simulink model "deney6"  (R2023b)
settings: Solver=VariableStepAuto  StartTime=0.0  StopTime=0.08  RelTol=1e-3
libraries: dspfdesign x1, commrandsrc3 x1, spsDiscreteVariableTimeDelayLib x1, commsink2 x1, commutil2 x1
settings Model: Creator=fatih  LastModifiedBy=fatih

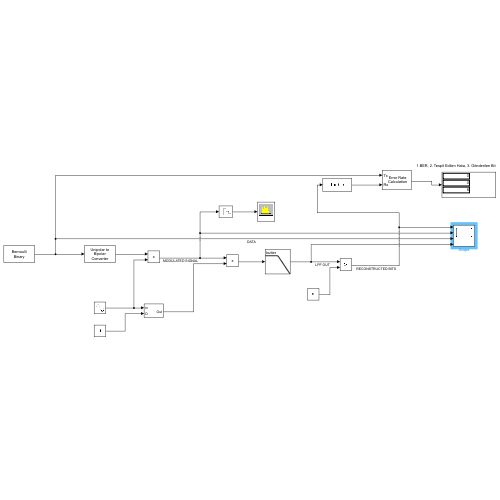
[thumbnail: Simulink's stored preview of the top-level diagram]
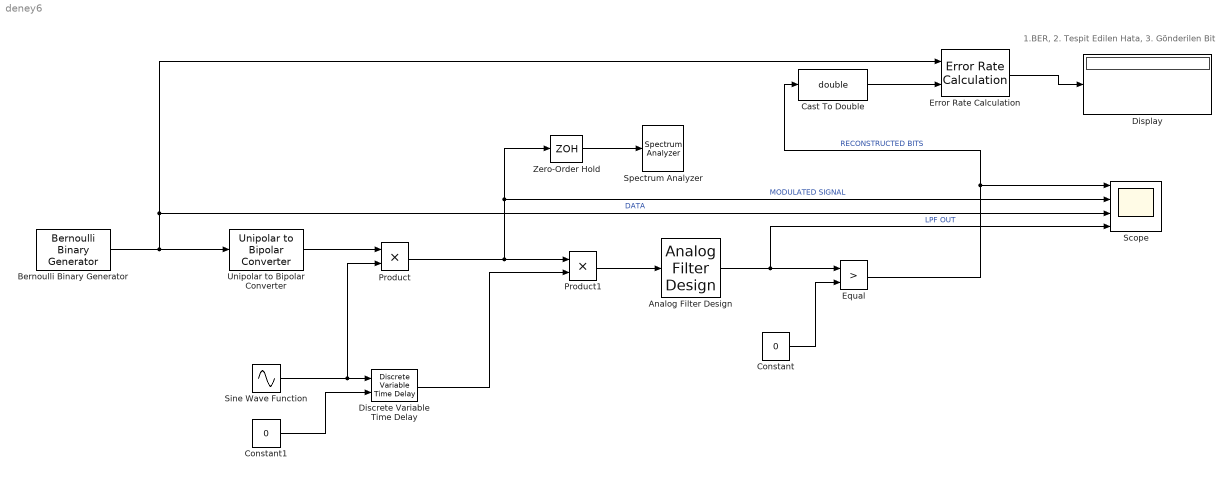
== system deney6 ==
  note: 1.BER, 2. Tespit Edilen Hata, 3. Gönderilen Bit
  Analog Filter Design : dspfdesign/Analog Filter Design  method=Butterworth  filttype=Lowpass  N=8  Wlo=2*pi*100  Whi=80  Rp=2  Rs=40
  Bernoulli Binary Generator : commrandsrc3/Bernoulli Binary Generator  ProbabilityOfZero=0.5  SeedSource=Auto  Seed=0  SampleTime=0.01  SamplesPerFrame=1  OutputDataType=double  SimulateUsing=Interpreted execution
  Cast To Double : DataTypeConversion  OutDataTypeStr=double  SaturateOnIntegerOverflow=off  RndMeth=Floor
  Constant : Constant  Value=0
  Constant1 : Constant  Value=0
  Discrete Variable Time Delay : spsDiscreteVariableTimeDelayLib/Discrete Variable Time Delay  MaxDelay=1  InitialValue=0  Ts=1e-5  DFT=on
      settings: LibrarySourceBlock=|
      | sps_lib/Control/Discrete Variable
      | Time Delay
  Display : Display
  Equal : RelationalOperator  Operator=>  OutDataTypeStr=boolean  RndMeth=Simplest  InputSameDT=off
  Error Rate Calculation : commsink2/Error Rate Calculation  N=1  st_delay=0  cp_mode=Entire frame  subframe=[]  PMode=Port  WsName=ErrorVec  RsMode2=off  stop=off  numErr=100  maxBits=1e6
      settings: LibrarySourceBlock=|
      | commhdlsink/Error Rate
      | Calculation
  Product : Product
  Product1 : Product
  Scope : Scope  NumInputPorts=4
  Sine Wave Function : Sin  Frequency=2*pi*1000  Phase=pi/2  SampleTime=1e-5
  Spectrum Analyzer : SpectrumAnalyzer  WindowPosition=[2.000000,372.000000,800.000000,500.000000,]  Visible=on  ScopeFrameLocation=window  Method=Welch  Span=99999.99999999999  StartFrequency=-49999.99999999999  StopFrequency=49999.99999999999  SpectrumUnits=Watts  FrequencyOffset=[0]  YLimits=[-0.01928317,0.1735529]
  Unipolar to Bipolar Converter : commutil2/Unipolar to Bipolar Converter  M=2  polarity=Positive  dataType=Inherit via internal rule
  Zero-Order Hold : ZeroOrderHold  SampleTime=-1
  wires:
  Bernoulli Binary Generator/1 -> Error Rate Calculation/1, Scope/3, Unipolar to Bipolar Converter/1  "DATA"
  Unipolar to Bipolar Converter/1 -> Product/1
  Sine Wave Function/1 -> Discrete Variable Time Delay/1, Product/2
  Product/1 -> Product1/1, Zero-Order Hold/1, Scope/2  "MODULATED SIGNAL"
  Product1/1 -> Analog Filter Design/1
  Constant/1 -> Equal/2
  Analog Filter Design/1 -> Scope/4, Equal/1  "LPF OUT"
  Cast To Double/1 -> Error Rate Calculation/2
  Error Rate Calculation/1 -> Display/1
  Equal/1 -> Cast To Double/1, Scope/1  "RECONSTRUCTED BITS"
  Zero-Order Hold/1 -> Spectrum Analyzer/1
  Discrete Variable Time Delay/1 -> Product1/2
  Constant1/1 -> Discrete Variable Time Delay/2
